simulink model "servo_motor_model"  (R2025b)
settings: Solver=VariableStepAuto  StartTime=0.0  StopTime=10.0  RelTol=1e-3
settings Model: Creator=youss  LastModifiedBy=youss

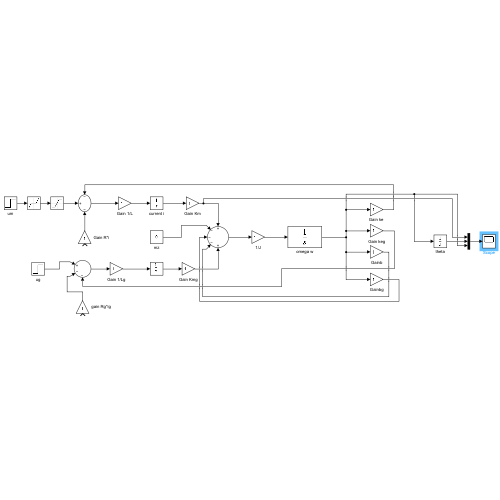
[thumbnail: Simulink's stored preview of the top-level diagram]
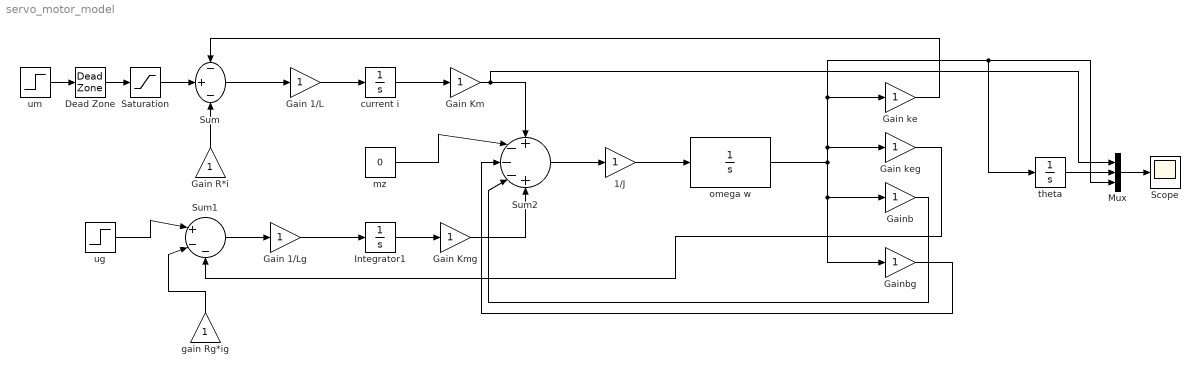
== system servo_motor_model ==
  1/J : Gain
  Dead Zone : DeadZone  LowerValue=-0.2  UpperValue=0.2
  Gain 1/L : Gain
  Gain 1/Lg : Gain
  Gain Km : Gain
  Gain Kmg : Gain
  Gain R*i : Gain
  "Gain ke " : Gain
  Gain keg : Gain
  Gainb : Gain
  Gainbg : Gain
  Integrator1 : Integrator
  Mux : Mux  Inputs=3
  Saturation : Saturate
  Scope : Scope
      settings: ActiveDisplayYMinimum=-1.8123553391376017  ActiveDisplayYMaximum=6.3123553391376026
  Sum : Sum  Inputs=-+-
  Sum1 : Sum  Inputs=|+--
  Sum2 : Sum  Inputs=+---+
  current i : Integrator
  gain Rg*ig : Gain
  mz : Constant  Value=0
  omega w : Integrator
  theta : Integrator
  ug : Step  Time=0  SampleTime=10
  um : Step  Time=0  SampleTime=10
  wires:
  um/1 -> Dead Zone/1
  Sum/1 -> Gain 1/L/1
  Gain 1/L/1 -> current i/1
  Gain R*i/1 -> Sum/3
  ug/1 -> Sum1/1
  Sum1/1 -> Gain 1/Lg/1
  Gain 1/Lg/1 -> Integrator1/1
  gain Rg*ig/1 -> Sum1/2
  current i/1 -> Gain Km/1
  Gain Km/1 -> Mux/1, Sum2/1
  Integrator1/1 -> Gain Kmg/1
  Gain Kmg/1 -> Sum2/5
  1/J/1 -> omega w/1
  Sum2/1 -> 1/J/1
  omega w/1 -> Mux/3, theta/1, "Gain ke "/1, Gain keg/1, Gainb/1, Gainbg/1
  "Gain ke "/1 -> Sum/1
  Gain keg/1 -> Sum1/3
  Gainb/1 -> Sum2/4
  Gainbg/1 -> Sum2/3
  mz/1 -> Sum2/2
  theta/1 -> Mux/2
  Mux/1 -> Scope/1
  Dead Zone/1 -> Saturation/1
  Saturation/1 -> Sum/2
